simulink model "Koniec"  (R2020b)
settings: Solver=VariableStepAuto  StartTime=0.0  StopTime=10.0  RelTol=1e-3
libraries: simulink x4
settings Model: Creator=jansz  LastModifiedBy=Krzysztof

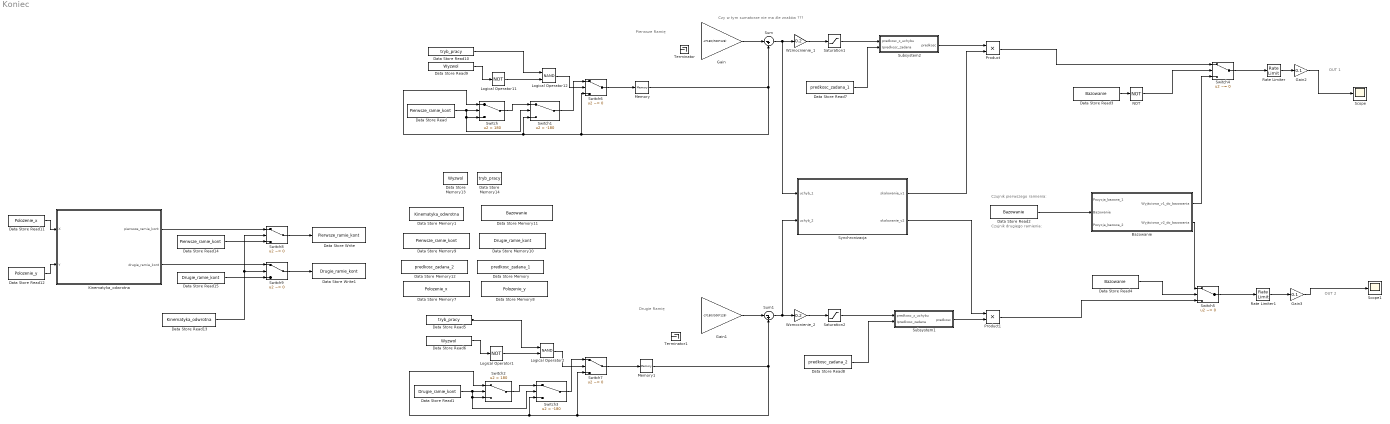
== system Koniec ==
  note: Czujnik drugiego ramienia:
  note: OUT 2
  note: Czy w tym sumatorze nie ma źle znaków ???
  note: Drugie Ramię
  note: Czujnik pierwszego ramienia:
  note: OUT 1
  note: Pierwsze Ramię
  Bazowanie : Subsystem
  Data Store Memory : DataStoreMemory  DataStoreName=predkosc_zadana_1  ReadBeforeWriteMsg=warning  WriteAfterWriteMsg=warning  WriteAfterReadMsg=warning  ShowAdditionalParam=off
  Data Store Memory1 : DataStoreMemory  DataStoreName=Kinematyka_odwrotna  ReadBeforeWriteMsg=warning  WriteAfterWriteMsg=warning  WriteAfterReadMsg=warning  ShowAdditionalParam=off
  Data Store Memory10 : DataStoreMemory  DataStoreName=Drugie_ramie_kont  ReadBeforeWriteMsg=warning  WriteAfterWriteMsg=warning  WriteAfterReadMsg=warning  ShowAdditionalParam=off
  Data Store Memory11 : DataStoreMemory  DataStoreName=Bazowanie  ReadBeforeWriteMsg=warning  WriteAfterWriteMsg=warning  WriteAfterReadMsg=warning  ShowAdditionalParam=off
  Data Store Memory12 : DataStoreMemory  DataStoreName=predkosc_zadana_2  ReadBeforeWriteMsg=warning  WriteAfterWriteMsg=warning  WriteAfterReadMsg=warning  ShowAdditionalParam=off
  Data Store Memory13 : DataStoreMemory  DataStoreName=Wyzwol  ReadBeforeWriteMsg=warning  WriteAfterWriteMsg=warning  WriteAfterReadMsg=warning  ShowAdditionalParam=off
  Data Store Memory14 : DataStoreMemory  DataStoreName=tryb_pracy  ReadBeforeWriteMsg=warning  WriteAfterWriteMsg=warning  WriteAfterReadMsg=warning  ShowAdditionalParam=off
  Data Store Memory7 : DataStoreMemory  DataStoreName=Polozenie_x  ReadBeforeWriteMsg=warning  WriteAfterWriteMsg=warning  WriteAfterReadMsg=warning  ShowAdditionalParam=off
  Data Store Memory8 : DataStoreMemory  DataStoreName=Polozenie_y  ReadBeforeWriteMsg=warning  WriteAfterWriteMsg=warning  WriteAfterReadMsg=warning  ShowAdditionalParam=off
  Data Store Memory9 : DataStoreMemory  DataStoreName=Pierwsze_ramie_kont  ReadBeforeWriteMsg=warning  WriteAfterWriteMsg=warning  WriteAfterReadMsg=warning  ShowAdditionalParam=off
  Data Store Read : DataStoreRead  DataStoreName=Pierwsze_ramie_kont
  Data Store Read1 : DataStoreRead  DataStoreName=Drugie_ramie_kont
  Data Store Read10 : DataStoreRead  DataStoreName=tryb_pracy
  Data Store Read11 : DataStoreRead  DataStoreName=Polozenie_x
  Data Store Read12 : DataStoreRead  DataStoreName=Polozenie_y
  Data Store Read13 : DataStoreRead  DataStoreName=Kinematyka_odwrotna
  Data Store Read14 : DataStoreRead  DataStoreName=Pierwsze_ramie_kont
  Data Store Read15 : DataStoreRead  DataStoreName=Drugie_ramie_kont
  Data Store Read2 : DataStoreRead  DataStoreName=Bazowanie
  Data Store Read3 : DataStoreRead  DataStoreName=Bazowanie
  Data Store Read4 : DataStoreRead  DataStoreName=Bazowanie
  Data Store Read5 : DataStoreRead  DataStoreName=tryb_pracy
  Data Store Read6 : DataStoreRead  DataStoreName=Wyzwol
  Data Store Read7 : DataStoreRead  DataStoreName=predkosc_zadana_1
  Data Store Read8 : DataStoreRead  DataStoreName=predkosc_zadana_2
  Data Store Read9 : DataStoreRead  DataStoreName=Wyzwol
  Data Store Write : DataStoreWrite  DataStoreName=Pierwsze_ramie_kont
  Data Store Write1 : DataStoreWrite  DataStoreName=Drugie_ramie_kont
  Gain : Gain  Gain=-2*180/(500*128)
  Gain1 : Gain  Gain=-2*180/(500*128)
  Gain2 : Gain  Gain=0.1
  Gain3 : Gain  Gain=0.1
  Kinematyka_odwrotna : Subsystem
  Logical Operator1 : Logic  Operator=NOT  AllPortsSameDT=off  OutDataTypeStr=boolean
  Logical Operator11 : Logic  Operator=NOT  AllPortsSameDT=off  OutDataTypeStr=boolean
  Logical Operator12 : Logic  Operator=NAND  AllPortsSameDT=off  OutDataTypeStr=boolean
  Logical Operator2 : Logic  Operator=NAND  AllPortsSameDT=off  OutDataTypeStr=boolean
  Memory : Memory
  Memory1 : Memory
  NOT : Logic  Operator=NOT  AllPortsSameDT=off  OutDataTypeStr=boolean
  Product : Product
  Product1 : Product
  Rate Limiter : RateLimiter  RisingSlewLimit=50  FallingSlewLimit=-50  SampleTimeMode=inherited
  Rate Limiter1 : RateLimiter  RisingSlewLimit=50  FallingSlewLimit=-50  SampleTimeMode=inherited
  Saturation1 : Saturate  UpperLimit=3  LowerLimit=-3
  Saturation2 : Saturate  UpperLimit=3  LowerLimit=-3
  Scope : Scope
  Scope1 : Scope
  Subsystem1 : Subsystem
  Subsystem2 : Subsystem
  Sum : Sum  Inputs=|-+
  Sum1 : Sum  Inputs=|-+
  Switch : Switch  Criteria=u2 > Threshold  Threshold=180
  Switch1 : Switch  Criteria=u2 > Threshold  Threshold=-180
  Switch2 : Switch  Criteria=u2 > Threshold  Threshold=180
  Switch3 : Switch  Criteria=u2 > Threshold  Threshold=-180
  Switch{4..9} (6 alike) : Switch  Criteria=u2 ~= 0
  Synchronizacja : Subsystem
  Terminator : Terminator
  Terminator1 : Terminator
  Wzmocnienie_1 : Gain  Gain=0.2
  Wzmocnienie_2 : Gain  Gain=0.2
  wires:
  Data Store Read11/1 -> Kinematyka_odwrotna/1(X)
  Data Store Read12/1 -> Kinematyka_odwrotna/2(Y)
  Data Store Read8/1 -> Subsystem1/2(Ipredkosc_zadana)
  Data Store Read10/1 -> Logical Operator12/1
  Subsystem2/1(predkosc) -> Product/1
  Switch6/1 -> Memory/1
  Data Store Read/1 -> Switch1/2, Switch/3, Switch/2
  Subsystem1/1(predkosc) -> Product1/2
  Switch4/1 -> Rate Limiter/1
  Data Store Read5/1 -> Logical Operator2/1
  Sum/1 -> Synchronizacja/1(uchyb_1), Wzmocnienie_1/1
  Switch1/1 -> Switch6/1
  Saturation2/1 -> Subsystem1/1(predkosc_z_uchybu)
  Gain2/1 -> Scope/1
  NOT/1 -> Switch4/2
  Data Store Read6/1 -> Logical Operator1/1
  Bazowanie/1(Wyjściowa_v1_do_bazowania) -> Switch4/3
  Sum1/1 -> Synchronizacja/2(uchyb_2), Wzmocnienie_2/1
  Data Store Read9/1 -> Logical Operator11/1
  Saturation1/1 -> Subsystem2/1(predkosc_z_uchybu)
  Rate Limiter/1 -> Gain2/1
  Rate Limiter1/1 -> Gain3/1
  Switch2/1 -> Switch3/1
  Switch7/1 -> Memory1/1
  Product/1 -> Switch4/1
  Wzmocnienie_1/1 -> Saturation1/1
  Data Store Read4/1 -> Switch5/2
  Logical Operator1/1 -> Logical Operator2/2
  Memory/1 -> Switch6/3, Switch1/3, Switch/1, Sum/2
  Gain1/1 -> Sum1/1
  Data Store Read7/1 -> Subsystem2/2(Ipredkosc_zadana)
  Logical Operator12/1 -> Switch6/2
  Bazowanie/2(Wyjściowa_v2_do_bazowania) -> Switch5/1
  Gain3/1 -> Scope1/1
  Switch/1 -> Switch1/1
  Data Store Read3/1 -> NOT/1
  Data Store Read2/1 -> Bazowanie/2(Bazowanie)
  Wzmocnienie_2/1 -> Saturation2/1
  Switch3/1 -> Switch7/1
  Memory1/1 -> Switch7/3, Switch3/3, Switch2/1, Sum1/2
  Data Store Read1/1 -> Switch3/2, Switch2/3, Switch2/2
  Synchronizacja/2(skalowanie_v2) -> Product1/1
  Product1/1 -> Switch5/3
  Logical Operator11/1 -> Logical Operator12/2
  Gain/1 -> Sum/1
  Logical Operator2/1 -> Switch7/2
  Switch5/1 -> Rate Limiter1/1
  Synchronizacja/1(skalowanie_v1) -> Product/2
  Kinematyka_odwrotna/1(pierwsze_ramie_kont) -> Switch8/1
  Kinematyka_odwrotna/2(drugie_ramie_kont) -> Switch9/1
  Data Store Read13/1 -> Switch8/2, Switch9/2
  Switch8/1 -> Data Store Write/1
  Switch9/1 -> Data Store Write1/1
  Data Store Read15/1 -> Switch9/3
  Data Store Read14/1 -> Switch8/3

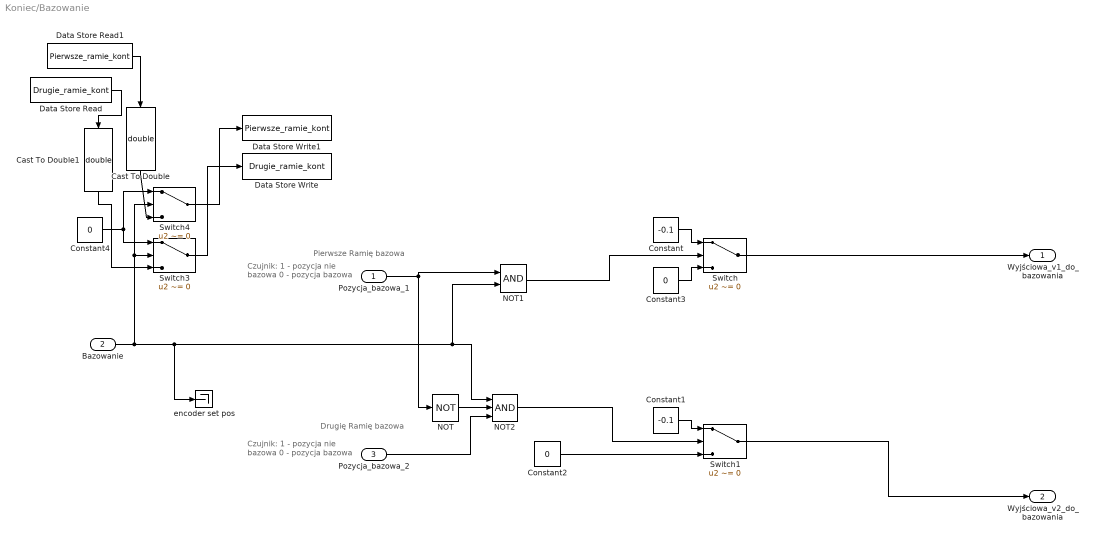
== system Koniec/Bazowanie ==
  note: Drugię Ramię bazowa
  note: Pierwsze Ramię bazowa
  note: Czujnik:
      | 1 - pozycja nie bazowa
      | 0 - pozycja bazowa
  note: Czujnik:
      | 1 - pozycja nie bazowa
      | 0 - pozycja bazowa
  Pozycja_bazowa_1 : Inport
  Bazowanie : Inport  Port=2
  Pozycja_bazowa_2 : Inport  Port=3
  Cast To Double : DataTypeConversion  OutDataTypeStr=double
  Cast To Double1 : DataTypeConversion  OutDataTypeStr=double
  Constant : Constant  Value=-0.1
  Constant1 : Constant  Value=-0.1
  Constant2 : Constant  Value=0
  Constant3 : Constant  Value=0
  Constant4 : Constant  Value=0
  Data Store Read : DataStoreRead  DataStoreName=Drugie_ramie_kont
  Data Store Read1 : DataStoreRead  DataStoreName=Pierwsze_ramie_kont
  Data Store Write : DataStoreWrite  DataStoreName=Drugie_ramie_kont
  Data Store Write1 : DataStoreWrite  DataStoreName=Pierwsze_ramie_kont
  NOT : Logic  Operator=NOT  AllPortsSameDT=off  OutDataTypeStr=boolean
  NOT1 : Logic  AllPortsSameDT=off  OutDataTypeStr=boolean
  NOT2 : Logic  Inputs=3  AllPortsSameDT=off  OutDataTypeStr=boolean
  Switch{,1,3..4} (4 alike) : Switch  Criteria=u2 ~= 0
  "encoder set pos " : Terminator
  Wyjściowa_v1_do_bazowania : Outport
  Wyjściowa_v2_do_bazowania : Outport  Port=2
  wires:
  Switch/1 -> Wyjściowa_v1_do_bazowania/1
  Pozycja_bazowa_1/1 -> NOT/1, NOT1/1
  Bazowanie/1 -> Switch4/2, Switch3/2, "encoder set pos "/1, NOT2/1, NOT1/2
  NOT1/1 -> Switch/2
  NOT2/1 -> Switch1/2
  Constant/1 -> Switch/1
  Constant1/1 -> Switch1/1
  Constant2/1 -> Switch1/3
  Constant3/1 -> Switch/3
  Pozycja_bazowa_2/1 -> NOT2/3
  NOT/1 -> NOT2/2
  Switch4/1 -> Data Store Write1/1
  Switch3/1 -> Data Store Write/1
  Data Store Read1/1 -> Cast To Double/1
  Cast To Double/1 -> Switch4/3
  Data Store Read/1 -> Cast To Double1/1
  Cast To Double1/1 -> Switch3/3
  Constant4/1 -> Switch3/1, Switch4/1
  Switch1/1 -> Wyjściowa_v2_do_bazowania/1

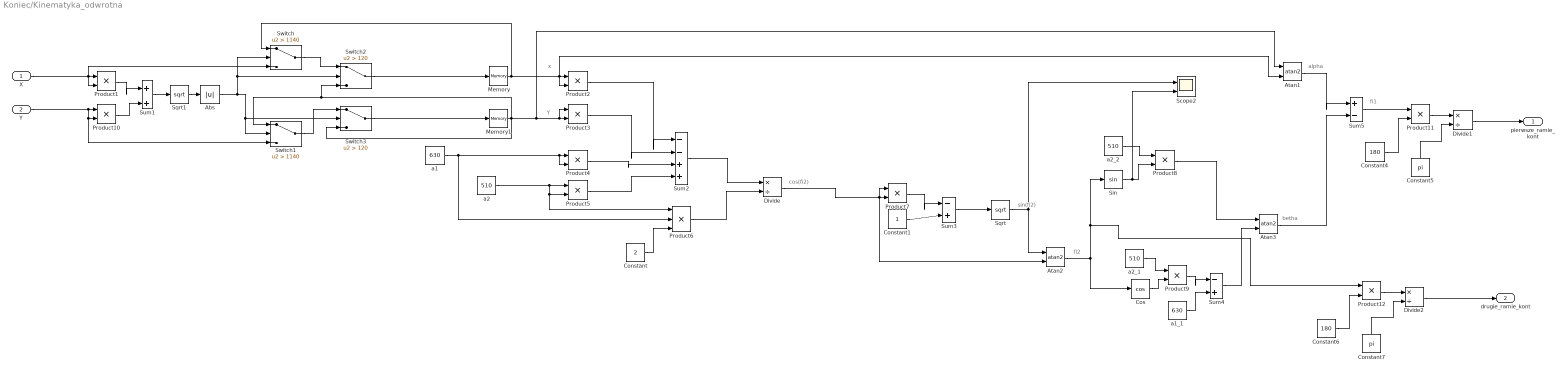
== system Koniec/Kinematyka_odwrotna ==
  note: betha
  note: fi2
  note: sin(fi2)
  note: cos(fi2)
  note: fi1
  note: alpha
  note: x
  note: Y
  X : Inport
  Y : Inport  Port=2
  Abs : Abs
  Atan1 : Trigonometry  Operator=atan2
  Atan2 : Trigonometry  Operator=atan2
  Atan3 : Trigonometry  Operator=atan2
  Constant : Constant  Value=2
  Constant1 : Constant
  Constant4 : Constant  Value=180
  Constant5 : Constant  Value=pi
  Constant6 : Constant  Value=180
  Constant7 : Constant  Value=pi
  Cos : Trigonometry  Operator=cos
  Divide : Product  Inputs=*/
  Divide1 : Product  Inputs=*/
  Divide2 : Product  Inputs=*/
  Memory : Memory
  Memory1 : Memory
  Product{1..5,7..12} (11 alike) : Product
  Product6 : Product  Inputs=3
  Scope2 : Scope  NumInputPorts=2
  Sin : Trigonometry
  Sqrt : Sqrt  SaturateOnIntegerOverflow=on
  Sqrt1 : Sqrt  SaturateOnIntegerOverflow=on
  Sum1 : Sum  Inputs=|++
  Sum2 : Sum  Inputs=|--++
  Sum3 : Sum  Inputs=|-+
  Sum4 : Sum  Inputs=|-+
  Sum5 : Sum  Inputs=|+-
  Switch : Switch  Criteria=u2 > Threshold  Threshold=1140
  Switch1 : Switch  Criteria=u2 > Threshold  Threshold=1140
  Switch2 : Switch  Criteria=u2 > Threshold  Threshold=120
  Switch3 : Switch  Criteria=u2 > Threshold  Threshold=120
  a1 : Constant  Value=630
  a1_1 : Constant  Value=630
  a2 : Constant  Value=510
  a2_1 : Constant  Value=510
  a2_2 : Constant  Value=510
  pierwsze_ramie_kont : Outport
  drugie_ramie_kont : Outport  Port=2
  wires:
  Constant/1 -> Product6/3
  a2/1 -> Product5/2, Product6/1, Product5/1
  a1/1 -> Product6/2, Product4/2, Product4/1
  Product7/1 -> Sum3/1
  Product5/1 -> Sum2/4
  Sqrt/1 -> Atan2/1, Scope2/1
  Product8/1 -> Atan3/1
  Sum4/1 -> Atan3/2
  Sum2/1 -> Divide/1
  Divide/1 -> Product7/1, Product7/2, Atan2/2
  a2_1/1 -> Product9/1
  Product3/1 -> Sum2/2
  Product4/1 -> Sum2/3
  Product2/1 -> Sum2/1
  Atan3/1 -> Sum5/2
  Product6/1 -> Divide/2
  Atan1/1 -> Sum5/1
  Sin/1 -> Scope2/2, Product8/2
  Constant1/1 -> Sum3/2
  a1_1/1 -> Sum4/2
  Sum3/1 -> Sqrt/1
  Product9/1 -> Sum4/1
  a2_2/1 -> Product8/1
  X/1 -> Switch/3, Product1/2, Product1/1
  Y/1 -> Switch1/3, Product10/2, Product10/1
  Product1/1 -> Sum1/1
  Product10/1 -> Sum1/2
  Sum1/1 -> Sqrt1/1
  Sqrt1/1 -> Abs/1
  Abs/1 -> Switch1/2, Switch3/2, Switch/2, Switch2/2
  Memory/1 -> Switch/1, Product2/2, Product2/1, Atan1/2
  Memory1/1 -> Switch3/3, Atan1/1, Product3/1, Product3/2, Switch2/3, Switch1/1
  Switch2/1 -> Memory/1
  Switch3/1 -> Memory1/1
  Switch1/1 -> Switch3/1
  Switch/1 -> Switch2/1
  Sum5/1 -> Product11/1
  Constant4/1 -> Product11/2
  Product11/1 -> Divide1/1
  Constant5/1 -> Divide1/2
  Divide1/1 -> pierwsze_ramie_kont/1
  Constant7/1 -> Divide2/2
  Atan2/1 -> Cos/1, Product12/1, Sin/1
  Constant6/1 -> Product12/2
  Product12/1 -> Divide2/1
  Divide2/1 -> drugie_ramie_kont/1
  Cos/1 -> Product9/2

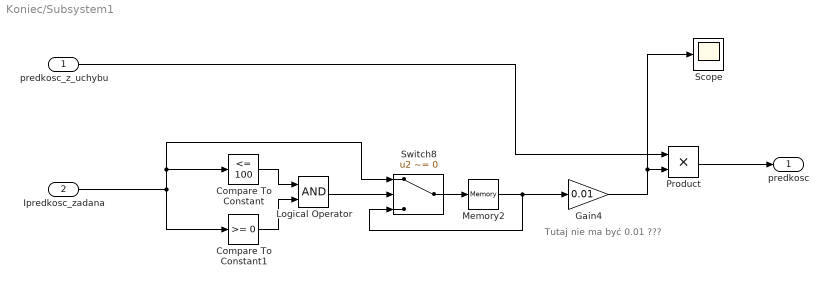
== system Koniec/Subsystem1 ==
  note: Tutaj nie ma być 0.01 ???
  predkosc_z_uchybu : Inport
  Ipredkosc_zadana : Inport  Port=2
  Compare To Constant : simulink/Logic and Bit Operations/Compare To Constant  relop=<=  const=100  OutDataTypeStr=boolean
  Compare To Constant1 : simulink/Logic and Bit Operations/Compare To Constant  relop=>=  const=0  OutDataTypeStr=boolean
  Gain4 : Gain  Gain=0.01
  Logical Operator : Logic  AllPortsSameDT=off  OutDataTypeStr=boolean
  Memory2 : Memory
  Product : Product
  Scope : Scope
  Switch8 : Switch  Criteria=u2 ~= 0
  predkosc : Outport
  wires:
  Compare To Constant1/1 -> Logical Operator/2
  Logical Operator/1 -> Switch8/2
  Compare To Constant/1 -> Logical Operator/1
  Product/1 -> predkosc/1
  Ipredkosc_zadana/1 -> Compare To Constant1/1, Switch8/1, Compare To Constant/1
  Memory2/1 -> Gain4/1, Switch8/3
  Gain4/1 -> Scope/1, Product/2
  predkosc_z_uchybu/1 -> Product/1
  Switch8/1 -> Memory2/1

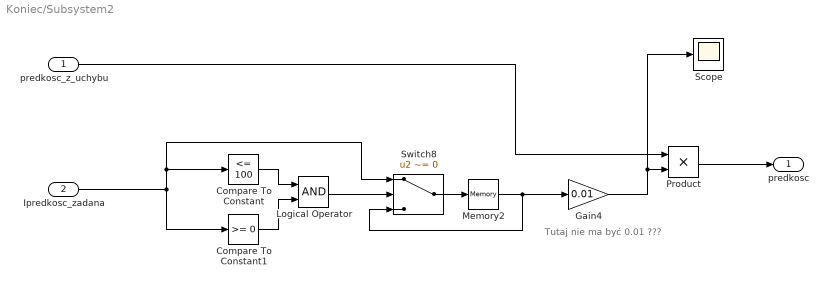
== system Koniec/Subsystem2 ==
  note: Tutaj nie ma być 0.01 ???
  predkosc_z_uchybu : Inport
  Ipredkosc_zadana : Inport  Port=2
  Compare To Constant : simulink/Logic and Bit Operations/Compare To Constant  relop=<=  const=100  OutDataTypeStr=boolean
  Compare To Constant1 : simulink/Logic and Bit Operations/Compare To Constant  relop=>=  const=0  OutDataTypeStr=boolean
  Gain4 : Gain  Gain=0.01
  Logical Operator : Logic  AllPortsSameDT=off  OutDataTypeStr=boolean
  Memory2 : Memory
  Product : Product
  Scope : Scope
  Switch8 : Switch  Criteria=u2 ~= 0
  predkosc : Outport
  wires:
  Compare To Constant1/1 -> Logical Operator/2
  Logical Operator/1 -> Switch8/2
  Compare To Constant/1 -> Logical Operator/1
  Product/1 -> predkosc/1
  Ipredkosc_zadana/1 -> Compare To Constant1/1, Switch8/1, Compare To Constant/1
  Memory2/1 -> Gain4/1, Switch8/3
  Gain4/1 -> Scope/1, Product/2
  predkosc_z_uchybu/1 -> Product/1
  Switch8/1 -> Memory2/1

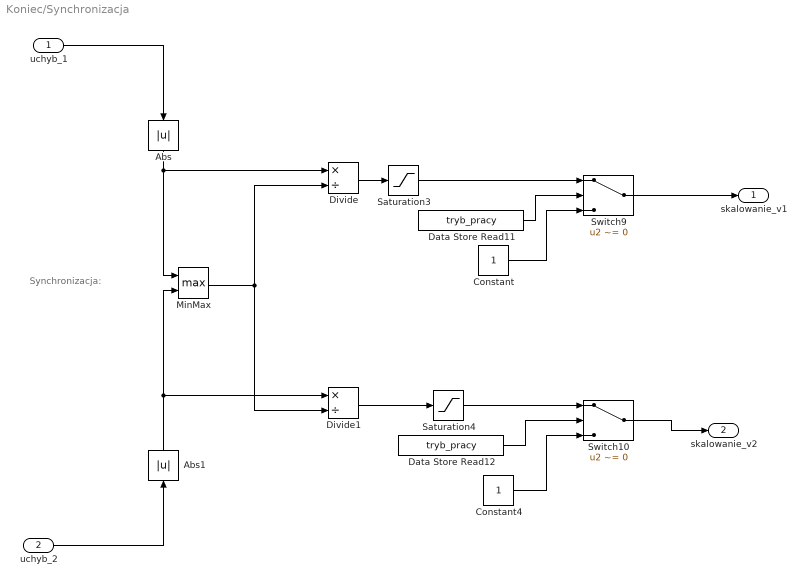
== system Koniec/Synchronizacja ==
  note: Synchronizacja:
  uchyb_1 : Inport
  uchyb_2 : Inport  Port=2
  Abs : Abs
  Abs1 : Abs
  Constant : Constant
  Constant4 : Constant
  Data Store Read11 : DataStoreRead  DataStoreName=tryb_pracy
  Data Store Read12 : DataStoreRead  DataStoreName=tryb_pracy
  Divide : Product  Inputs=*/
  Divide1 : Product  Inputs=*/
  MinMax : MinMax  Function=max  Inputs=2
  Saturation3 : Saturate  UpperLimit=1  LowerLimit=0.001
  Saturation4 : Saturate  UpperLimit=1  LowerLimit=0.001
  Switch10 : Switch  Criteria=u2 ~= 0
  Switch9 : Switch  Criteria=u2 ~= 0
  skalowanie_v1 : Outport
  skalowanie_v2 : Outport  Port=2
  wires:
  Abs/1 -> Divide/1, MinMax/1
  Abs1/1 -> MinMax/2, Divide1/1
  Data Store Read11/1 -> Switch9/2
  uchyb_2/1 -> Abs1/1
  MinMax/1 -> Divide1/2, Divide/2
  Constant/1 -> Switch9/3
  Constant4/1 -> Switch10/3
  Switch9/1 -> skalowanie_v1/1
  Saturation4/1 -> Switch10/1
  uchyb_1/1 -> Abs/1
  Data Store Read12/1 -> Switch10/2
  Saturation3/1 -> Switch9/1
  Divide/1 -> Saturation3/1
  Divide1/1 -> Saturation4/1
  Switch10/1 -> skalowanie_v2/1
